simulink library "SynapsesLib"  (Simulink 7.7)
settings: Solver=ode45  SolverMode=SingleTasking  StartTime=0.0  StopTime=10.0  RelTol=1e-3
undefined symbols (not defined in the file or in its folder): EAmpa, FTampa, gAmpa, RTampa
libraries: WaveformsLib x7, CurrentsLib x7, SynapsesLib x1
settings Model: Creator=jpalma  LastModifiedBy=jpalma

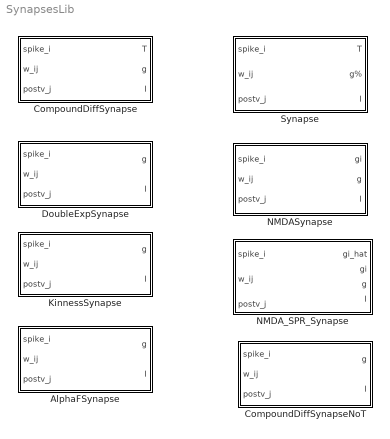
== system SynapsesLib ==
  AlphaFSynapse : Subsystem  mask{EZ=0, gZ=1, tauZ=10}
      mask prompts: EZ "Eq Voltage, EZ"; gZ "Conductance, gZ"; tauZ "Decay Time, tauZ"
      mask help: Author: Jesse Palma
      mask Help: Author: Jesse Palma
      mask Display: image(imread('../Libs/icons/Synapse.jpg'),'center');
  CompoundDiffSynapse : Subsystem  mask{EZ=EAmpa, gZ=gAmpa, tauRZ=RTampa, tauFZ=FTampa}
      mask prompts: EZ "Eq Voltage, EZ"; gZ "Conductance, gZ"; tauRZ "Rise Time, tauRZ"; tauFZ "Fall Time, tauFZ"
      mask help: Author: Jesse Palma
      mask Help: Author: Jesse Palma
      mask Display: image(imread('../Libs/icons/Synapse.jpg'),'center');
  CompoundDiffSynapseNoT : Subsystem  mask{EZ=EAmpa, gZ=gAmpa, tauRZ=RTampa, tauFZ=FTampa}
      mask prompts: EZ "Eq Voltage, EZ"; gZ "Conductance, gZ"; tauRZ "Rise Time, tauRZ"; tauFZ "Fall Time, tauFZ"
      mask help: Author: Jesse Palma
      mask Help: Author: Jesse Palma
      mask Display: image(imread('../Libs/icons/Synapse.jpg'),'center');
  DoubleExpSynapse : Subsystem  mask{EZ=EAmpa, gZ=gAmpa, tauRZ=RTampa, tauFZ=FTampa}
      mask prompts: EZ "Eq Voltage, EZ"; gZ "Conductance, gZ"; tauRZ "Rise Time, tauRZ"; tauFZ "Fall Time, tauFZ"
      mask help: Author: Jesse Palma
      mask Help: Author: Jesse Palma
      mask Display: image(imread('../Libs/icons/Synapse.jpg'),'center');
  KinnessSynapse : Subsystem  mask{EZ=EAmpa, gZ=gAmpa, tauRZ=RTampa, tauFZ=FTampa}
      mask prompts: EZ "Eq Voltage, EZ"; gZ "Conductance, gZ"; tauRZ "Rise Time, tauRZ"; tauFZ "Fall Time, tauFZ"
      mask help: Author: Jesse Palma
      mask Help: Author: Jesse Palma
      mask Display: image(imread('../Libs/icons/Synapse.jpg'),'center');
  NMDASynapse : Subsystem  mask{EZ=0, gZ=0.005, tauRZ=0.33, tauFZ=40, etaZ=0.33, mgZ=1, gammaZ=0.06, gainZ=4}
      mask prompts: EZ "Eq Voltage, EZ"; gZ "Conductance, gZ"; tauRZ "Rise Time, tauRZ"; tauFZ "Fall Time, tauFZ"; etaZ "Voltage-dependence, etaZ"; mgZ "Mg concentration, mgZ"; gammaZ "Voltage-chandge-dependence, gammaZ"; gainZ "Concentration Gain, gN"
      mask help: Author: Jesse Palma
      mask Help: Author: Jesse Palma
      mask Display: image(imread('../Libs/icons/Synapse.jpg'),'center');
  NMDA_SPR_Synapse : Subsystem  mask{EZ=0, gZ=0.005, tauRZ=0.33, tauFZ=40, etaZ=0.33, mgZ=1, gammaZ=0.06, gainZ=4}
      mask prompts: EZ "Eq Voltage, EZ"; gZ "Conductance, gZ"; tauRZ "Rise Time, tauRZ"; tauFZ "Fall Time, tauFZ"; etaZ "Voltage-dependence, etaZ"; mgZ "Mg concentration, mgZ"; gammaZ "Voltage-chandge-dependence, gammaZ"; gainZ "Concentration Gain, gN"
      mask help: Author: Jesse Palma
      mask Help: Author: Jesse Palma
      mask Display: image(imread('../Libs/icons/Synapse.jpg'),'center');
  Synapse : Subsystem  BlockChoice=CompoundDiffSynapse
      settings: TemplateBlock=self  MemberBlocks=CompoundDiffSynapse,DoubleExpSynapse,KinnessSynapse
      mask Display: image(imread('../Libs/icons/Synapse.jpg'),'center');

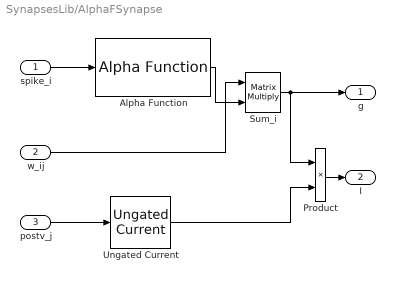
== system SynapsesLib/AlphaFSynapse ==
  spike_i : Inport
  w_ij : Inport  Port=2
  postv_j : Inport  Port=3
  Alpha Function : WaveformsLib/Alpha Function  SystemSampleTime=-1  tauDecay=tauZ  onsetStr=1
  Product : Product  RndMeth=Zero
  Sum_i : Product  Multiplication=Matrix(*)
  Ungated Current : CurrentsLib/Ungated Current  SystemSampleTime=-1  EX=EZ  gX=gZ
  g : Outport
  I : Outport  Port=2
  wires:
  Product/1 -> I/1
  spike_i/1 -> Alpha Function/1
  Ungated Current/1 -> Product/2
  postv_j/1 -> Ungated Current/1
  Sum_i/1 -> Product/1, g/1
  Alpha Function/1 -> Sum_i/2
  w_ij/1 -> Sum_i/1

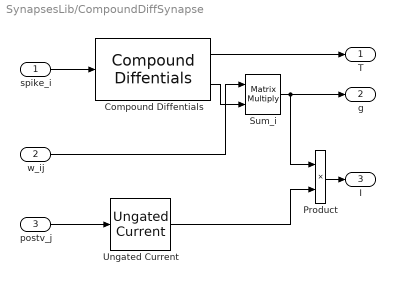
== system SynapsesLib/CompoundDiffSynapse ==
  spike_i : Inport
  w_ij : Inport  Port=2
  postv_j : Inport  Port=3
  Compound Diffentials : WaveformsLib/Compound Diffentials  SystemSampleTime=-1  tauRise=tauRZ  tauFall=tauFZ  squareWaveWidth=tauRZ  squareWaveHeight=1/tauRZ  interGain=2/tauRZ  finalGain=(tauFZ+tauRZ)/tauFZ
  Product : Product  RndMeth=Zero
  Sum_i : Product  Multiplication=Matrix(*)
  Ungated Current : CurrentsLib/Ungated Current  SystemSampleTime=-1  EX=EZ  gX=gZ
  T : Outport
  g : Outport  Port=2
  I : Outport  Port=3
  wires:
  Product/1 -> I/1
  spike_i/1 -> Compound Diffentials/1
  Ungated Current/1 -> Product/2
  Compound Diffentials/1 -> T/1
  postv_j/1 -> Ungated Current/1
  Sum_i/1 -> Product/1, g/1
  Compound Diffentials/2 -> Sum_i/2
  w_ij/1 -> Sum_i/1

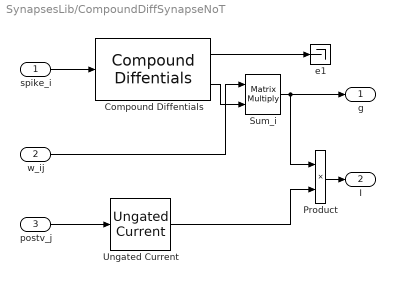
== system SynapsesLib/CompoundDiffSynapseNoT ==
  spike_i : Inport
  w_ij : Inport  Port=2
  postv_j : Inport  Port=3
  Compound Diffentials : WaveformsLib/Compound Diffentials  SystemSampleTime=-1  tauRise=tauRZ  tauFall=tauFZ  squareWaveWidth=tauRZ  squareWaveHeight=1/tauRZ  interGain=2/tauRZ  finalGain=(tauFZ+tauRZ)/tauFZ
  Product : Product  RndMeth=Zero
  Sum_i : Product  Multiplication=Matrix(*)
  Ungated Current : CurrentsLib/Ungated Current  SystemSampleTime=-1  EX=EZ  gX=gZ
  e1 : Terminator
  g : Outport
  I : Outport  Port=2
  wires:
  Product/1 -> I/1
  spike_i/1 -> Compound Diffentials/1
  Ungated Current/1 -> Product/2
  postv_j/1 -> Ungated Current/1
  Sum_i/1 -> Product/1, g/1
  Compound Diffentials/2 -> Sum_i/2
  w_ij/1 -> Sum_i/1
  Compound Diffentials/1 -> e1/1

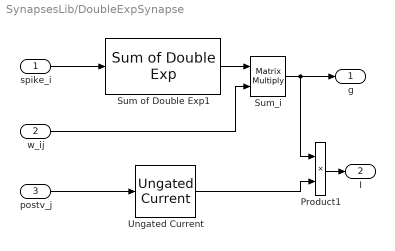
== system SynapsesLib/DoubleExpSynapse ==
  spike_i : Inport
  w_ij : Inport  Port=2
  postv_j : Inport  Port=3
  Product1 : Product  RndMeth=Zero
  Sum of Double Exp1 : WaveformsLib/Sum of Double Exp  SystemSampleTime=-1  tauRise=tauRZ  tauFall=tauFZ  timeStep=0.01
  Sum_i : Product  Multiplication=Matrix(*)
  Ungated Current : CurrentsLib/Ungated Current  SystemSampleTime=-1  EX=EZ  gX=gZ
  g : Outport
  I : Outport  Port=2
  wires:
  Product1/1 -> I/1
  spike_i/1 -> Sum of Double Exp1/1
  Ungated Current/1 -> Product1/2
  postv_j/1 -> Ungated Current/1
  Sum of Double Exp1/1 -> Sum_i/1
  w_ij/1 -> Sum_i/2
  Sum_i/1 -> g/1, Product1/1

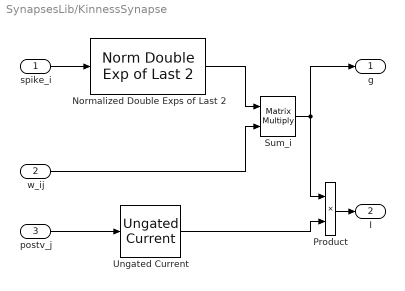
== system SynapsesLib/KinnessSynapse ==
  spike_i : Inport
  w_ij : Inport  Port=2
  postv_j : Inport  Port=3
  Normalized Double Exps of Last 2 : WaveformsLib/Norm Double Exp of Last 2  SystemSampleTime=-1  tauRise=tauR  tauFall=tauF
  Product : Product  RndMeth=Zero
  Sum_i : Product  Multiplication=Matrix(*)
  Ungated Current : CurrentsLib/Ungated Current  SystemSampleTime=-1  EX=EZ  gX=gZ
  g : Outport
  I : Outport  Port=2
  wires:
  Product/1 -> I/1
  spike_i/1 -> Normalized Double Exps of Last 2/1
  Ungated Current/1 -> Product/2
  postv_j/1 -> Ungated Current/1
  Normalized Double Exps of Last 2/1 -> Sum_i/1
  Sum_i/1 -> g/1, Product/1
  w_ij/1 -> Sum_i/2

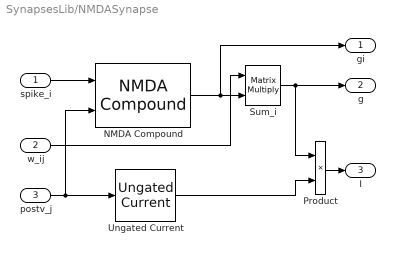
== system SynapsesLib/NMDASynapse ==
  spike_i : Inport
  w_ij : Inport  Port=2
  postv_j : Inport  Port=3
  NMDA Compound : WaveformsLib/NMDA Compound  SystemSampleTime=-1  rt=tauRZ  ft=tauFZ  eta=etaZ  mg=mgZ  gamma=gammaZ  gn=gainZ
  Product : Product  RndMeth=Zero
  Sum_i : Product  Multiplication=Matrix(*)
  Ungated Current : CurrentsLib/Ungated Current  SystemSampleTime=-1  EX=EZ  gX=gZ
  gi : Outport
  g : Outport  Port=2
  I : Outport  Port=3
  wires:
  w_ij/1 -> Sum_i/1
  NMDA Compound/1 -> Sum_i/2, gi/1
  Sum_i/1 -> g/1, Product/1
  postv_j/1 -> Ungated Current/1, NMDA Compound/2
  Ungated Current/1 -> Product/2
  spike_i/1 -> NMDA Compound/1
  Product/1 -> I/1

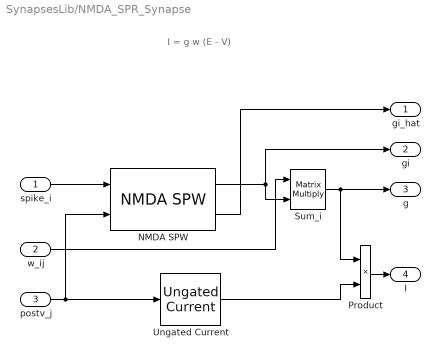
== system SynapsesLib/NMDA_SPR_Synapse ==
  note: I = g w (E - V)
  spike_i : Inport
  w_ij : Inport  Port=2
  postv_j : Inport  Port=3
  NMDA SPW : WaveformsLib/NMDA SPW  SystemSampleTime=-1  trise=tauRZ  tfall=tauFZ  eta=etaZ  mg=mgZ  gamma=gammaZ  gn=gainZ
  Product : Product  RndMeth=Zero
  Sum_i : Product  Multiplication=Matrix(*)
  Ungated Current : CurrentsLib/Ungated Current  SystemSampleTime=-1  EX=EZ  gX=gZ
  gi_hat : Outport
  gi : Outport  Port=2
  g : Outport  Port=3
  I : Outport  Port=4
  wires:
  Product/1 -> I/1
  spike_i/1 -> NMDA SPW/1
  Ungated Current/1 -> Product/2
  postv_j/1 -> Ungated Current/1, NMDA SPW/2
  Sum_i/1 -> Product/1, g/1
  NMDA SPW/1 -> gi/1, Sum_i/2
  w_ij/1 -> Sum_i/1
  NMDA SPW/2 -> gi_hat/1

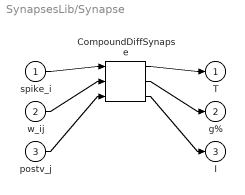
== system SynapsesLib/Synapse ==
  spike_i : Inport
  w_ij : Inport  Port=2
  postv_j : Inport  Port=3
  CompoundDiffSynapse : SynapsesLib/CompoundDiffSynapse  SystemSampleTime=-1  EZ=EAmpa  gZ=gAmpa  tauRZ=RTampa  tauFZ=FTampa
  T : Outport
  g% : Outport  Port=2
  I : Outport  Port=3
  wires:
  spike_i/1 -> CompoundDiffSynapse/1
  w_ij/1 -> CompoundDiffSynapse/2
  postv_j/1 -> CompoundDiffSynapse/3
  CompoundDiffSynapse/1 -> T/1
  CompoundDiffSynapse/2 -> g%/1
  CompoundDiffSynapse/3 -> I/1
